simulink model "Maths_Eqn_2"  (R2022b)
settings: Solver=VariableStepAuto  StartTime=0.0  StopTime=10.0  RelTol=1e-3
model workspace (MAT data in the model file):
  u = Simulink.Parameter
  u.DataType = 'auto'
  u.Complexity = 'real'
  u.Dimensions = [0 0]
  x = Simulink.Parameter
  x.DataType = 'auto'
  x.Complexity = 'real'
  x.Dimensions = [0 0]
libraries: simulink x1
settings Model: Creator=Ayush Pharande  LastModifiedBy=Ayush Pharande

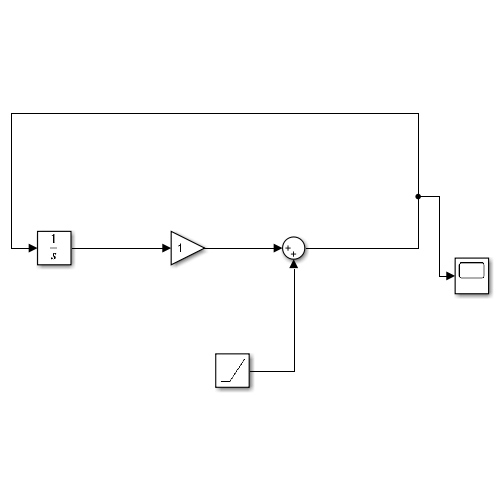
[thumbnail: Simulink's stored preview of the top-level diagram]
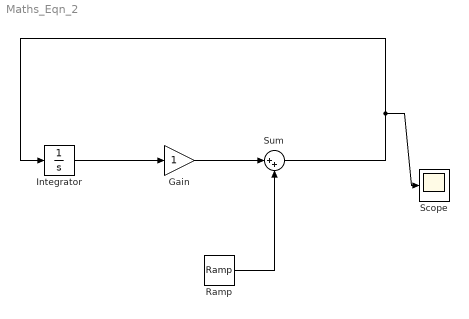
== system Maths_Eqn_2 ==
  Gain : Gain
  Integrator : Integrator
  Ramp : simulink/Sources/Ramp  slope=1  start=0  InitialOutput=0
  Scope : Scope
  Sum : Sum  Inputs=|++
  wires:
  Integrator/1 -> Gain/1
  Gain/1 -> Sum/1
  Sum/1 -> Integrator/1, Scope/1
  Ramp/1 -> Sum/2
